simulink model "secondSimulink"  (R2017a)
settings: Solver=VariableStepAuto  StartTime=0.0  StopTime=10.0  RelTol=1e-3
libraries: simulink x4
settings Model: Creator=Pc  LastModifiedBy=Pc

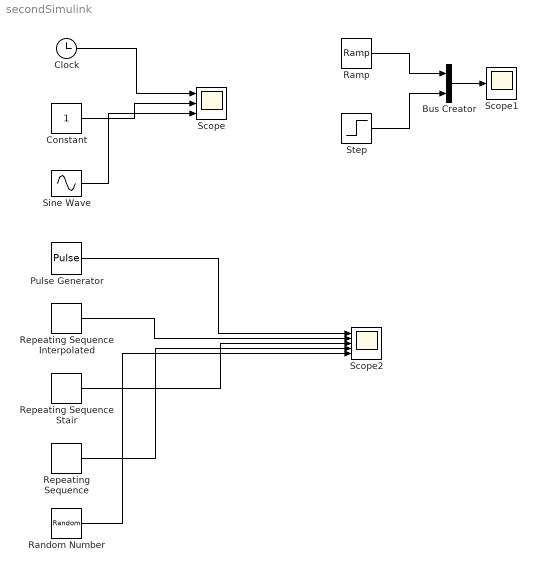
== system secondSimulink ==
  Bus Creator : BusCreator  Inputs=2
  Clock : Clock
  Constant : Constant
  Pulse Generator : DiscretePulseGenerator  PulseType=Time based  Period=10  PulseWidth=5
  Ramp : simulink/Sources/Ramp  slope=1  start=0  X0=0
  Random Number : RandomNumber  SampleTime=0.1
  Repeating Sequence : simulink/Sources/Repeating Sequence  rep_seq_t=[0 2]  rep_seq_y=[0 2]
  Repeating Sequence Interpolated : simulink/Sources/Repeating Sequence Interpolated  OutValues=[3 1 4 2 1].'  TimeValues=[0 0.1 0.5 0.6 1].'  LookUpMeth=Interpolation-Use End Values  tsamp=0.01  OutMin=[]  OutMax=[]  OutDataTypeStr=double  OutputDataTypeScalingMode=double  OutDataType=fixdt(0,8)  OutScaling=2^-10
  Repeating Sequence Stair : simulink/Sources/Repeating Sequence Stair  OutValues=[3 1 4 2 1].'  tsamp=-1  OutMin=[]  OutMax=[]  OutDataTypeStr=double  OutputDataTypeScalingMode=double  OutDataType=fixdt(0,8)  ConRadixGroup=Best Precision: Vector-wise  OutScaling=2^-12
  Scope : Scope  NumInputPorts=3
  Scope1 : Scope
  Scope2 : Scope  NumInputPorts=5
  Sine Wave : Sin  SampleTime=0
  Step : Step  SampleTime=0
  wires:
  Clock/1 -> Scope/1
  Constant/1 -> Scope/2
  Sine Wave/1 -> Scope/3
  Ramp/1 -> Bus Creator/1
  Step/1 -> Bus Creator/2
  Bus Creator/1 -> Scope1/1
  Pulse Generator/1 -> Scope2/1
  Repeating Sequence Interpolated/1 -> Scope2/2
  Repeating Sequence Stair/1 -> Scope2/3
  Repeating Sequence/1 -> Scope2/4
  Random Number/1 -> Scope2/5
